simulink subsystem "MyMPC"  (R2020b)
settings: Solver=VariableStepAuto  StartTime=0.0  StopTime=10.0  RelTol=1e-3
values from neighbouring files (symbols this model uses):
  A = d_sys.A    [MPC_Init.m]    (also in init.m = [a11 a12 0 0;     a21 a22 0 0;     0 1 0 0;     v ls v 0])
  B = d_sys.B    [MPC_Init.m]    (also in init.m = [2*cf/(m*v) 0; 2*lf*cf/iz 0; 0 -v ;0  0])
  C = d_sys.C    [MPC_Init.m]    (also in init.m = [0 0 1 0; 0 0 0 1])
  L = place(A',C',kl)    [init.m]
undefined symbols (not defined in the file or in its folder): DiscIntNeverNeededParam, PredictionHorizon
settings Model: Creator=Stage  LastModifiedBy=Stage

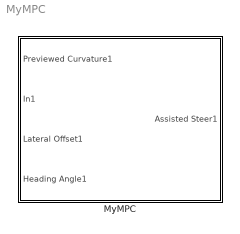
== system MyMPC ==
  MyMPC : Subsystem

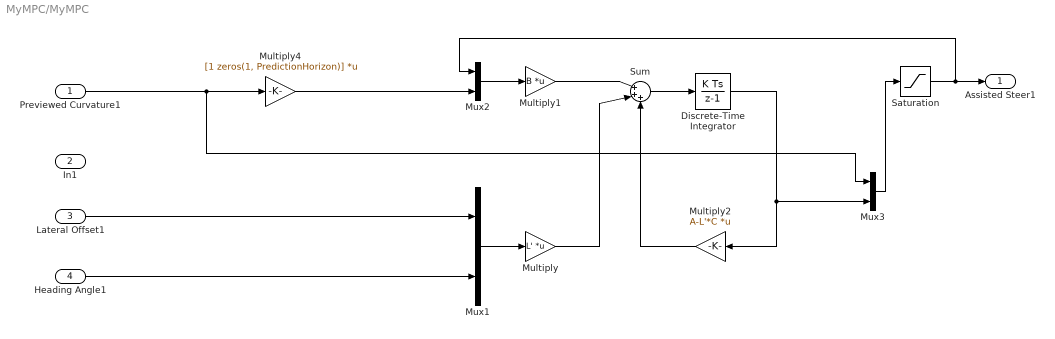
== system MyMPC/MyMPC ==
  Previewed Curvature1 : Inport
  In1 : Inport  Port=2
  Lateral Offset1 : Inport  Port=3
  Heading Angle1 : Inport  Port=4
  Discrete-Time Integrator : DiscreteIntegrator  SampleTime=-1  ICPrevOutput=DiscIntNeverNeededParam  ICPrevScaledInput=DiscIntNeverNeededParam
  Multiply : Gain  Gain=L'  Multiplication=Matrix(K*u) (u vector)
  Multiply1 : Gain  Gain=B  Multiplication=Matrix(K*u) (u vector)
  Multiply2 : Gain  Gain=A-L'*C  Multiplication=Matrix(K*u) (u vector)
  Multiply4 : Gain  Gain=[1 zeros(1, PredictionHorizon)]  Multiplication=Matrix(K*u) (u vector)
  Mux1 : Mux  Inputs=2
  Mux2 : Mux  Inputs=2
  Mux3 : Mux  Inputs=2
  Saturation : Saturate  UpperLimit=0.2  LowerLimit=-0.2
  Sum : Sum  Inputs=|+++
  Assisted Steer1 : Outport
  wires:
  Saturation/1 -> Mux2/1, Assisted Steer1/1
  Multiply1/1 -> Sum/1
  Discrete-Time Integrator/1 -> Mux3/2, Multiply2/1
  Mux2/1 -> Multiply1/1
  Multiply/1 -> Sum/2
  Mux3/1 -> Saturation/1
  Lateral Offset1/1 -> Mux1/1
  Heading Angle1/1 -> Mux1/2
  Previewed Curvature1/1 -> Mux3/1, Multiply4/1
  Sum/1 -> Discrete-Time Integrator/1
  Multiply4/1 -> Mux2/2
  Mux1/1 -> Multiply/1
  Multiply2/1 -> Sum/3
